simulink model "power_distline"  (Simulink 6.0)
settings: Solver=ode15s  SolverMode=SingleTasking  StartTime=0.0  StopTime=0.1  MaxStep=50e-6  RelTol=1e-3  AbsTol=1e-6
libraries: powerlib x10
settings Model: Creator=patrice  LastModifiedBy=batserve  ExtModeTrigMode=oneshot  ExtModeArmWhenConnect=off  ExtModeAutoUpdateStatusClock=off
settings DataIOCC: LimitDataPoints=off  SignalLoggingName=sigsOut
settings OptimizationCC: BooleanDataType=off
settings DebuggingCC: SolverPrmCheckMsg=none
settings HardwareCC: TargetUnknown=on
settings RTWCC: TemplateMakefile=grt_unix.tmf

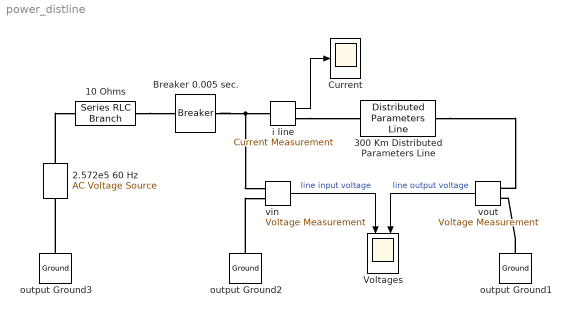
== system power_distline ==
  10 Ohms : powerlib/Elements/Series RLC Branch  PhysicalDomain=powersysdomain  SubClassName=unknown  LeftPortType=p1  RightPortType=p1  LConnTagsString=__new0  RConnTagsString=__new0  Resistance=10  Inductance=0  Capacitance=inf  Measurements=None
  "2.572e5 60 Hz " : powerlib/Electrical Sources/AC Voltage Source  Description=source block  Orientation=up  Amplitude=(315e3*sqrt(2))/sqrt(30)  Phase=0  Frequency=60  SampleTime=0  Measurements=None
      settings: AttributesFormatString=\n
  300 Km Distributed Parameters Line : powerlib/Elements/Distributed Parameters Line  Phases=1  Frequency=60  Resistance=0.2568  Inductance=2.0e-3  Capacitance=8.6e-9  Length=300  x1=[0 -1.992e-09;0.0002737 -2.609e-09;0.0005474 -3.197e-09;0.0008212 -3.752e-09;0.001095 -4.267e-09;0.001369 -4.736e-09]  x2=[0 -1.992e-09;0.0002737 -2.609e-09;0.0005474 -3.197e-09;0.0008212 -3.752e-09;0.001095 -4.267e-09;0.001369 -4.736e-09]  x3=[0 -8.754e-13;0.0002737 -2.116e-12;0.0005474 -3.334e-12;0.0008212 -4.517e-12;0.001095 -5.651e-12;0.001369 -6.726e-12]  x4=[0 -8.754e-13;0.0002737 -2.116e-12;0.0005474 -3.334e-12;0.0008212 -4.517e-12;0.001095 -5.651e-12;0.001369 -6.726e-12]  x5=0.001369  Measurements=None
      settings: AttributesFormatString=\n
  Breaker 0.005 sec. : powerlib/Elements/Breaker  BreakerResistance=1e-1  InitialState=0  SnubberResistance=inf  SnubberCapacitance=0  SwitchingTimes=[ .005 ]  External=off  Measurements=None
      settings: AttributesFormatString=\n
  Current : Scope
      settings: TickLabels=on  TimeRange=0.05  YMin=-100000  YMax=100000  DataFormat=Array
  Voltages : Scope  NumInputPorts=2
      settings: Orientation=down  TickLabels=on  TimeRange=0.1  YMin=-100000~-200000  YMax=100000~200000  DataFormat=Array  MaxDataPoints=5000000
  i line : powerlib/Measurements/Current Measurement  Tag=PoWeRsYsTeMmEaSuReMeNt  PhasorSimulation=off  OutputType=Magnitude  PSBequivalent=0
  output Ground1 : powerlib/Elements/Ground  Orientation=down  PhysicalDomain=powersysdomain  SubClassName=unknown  LeftPortType=p1  RightPortType=p1  LConnTagsString=a  RConnTagsString=__newr0
  output Ground2 : powerlib/Elements/Ground  Orientation=down  PhysicalDomain=powersysdomain  SubClassName=unknown  LeftPortType=p1  RightPortType=p1  LConnTagsString=a  RConnTagsString=__newr0
  output Ground3 : powerlib/Elements/Ground  Orientation=down  PhysicalDomain=powersysdomain  SubClassName=unknown  LeftPortType=p1  RightPortType=p1  LConnTagsString=a  RConnTagsString=__newr0
  vin : powerlib/Measurements/Voltage Measurement  Tag=PoWeRsYsTeMmEaSuReMeNt  PhasorSimulation=off  OutputType=Magnitude  PSBequivalent=0
  vout : powerlib/Measurements/Voltage Measurement  Tag=PoWeRsYsTeMmEaSuReMeNt  Orientation=left  PhasorSimulation=off  OutputType=Magnitude  PSBequivalent=0
  wires:
  i line/1 -> Current/1
  vin/1 -> Voltages/1  "line input voltage"
  vout/1 -> Voltages/2  "line output voltage"
  connections:
  output Ground2/LConn1 -- vin/LConn2
  Breaker 0.005 sec./RConn1 -- vin/LConn1 -- i line/LConn1
  "2.572e5 60 Hz "/RConn1 -- 10 Ohms/LConn1
  10 Ohms/RConn1 -- Breaker 0.005 sec./LConn1
  output Ground3/LConn1 -- "2.572e5 60 Hz "/LConn1
  i line/RConn1 -- 300 Km Distributed Parameters Line/LConn1
  300 Km Distributed Parameters Line/RConn1 -- vout/LConn1
  output Ground1/LConn1 -- vout/LConn2
